simulink model "l512_devel_pps_2016f"  (R2012b)
settings: Solver=ode45  StartTime=0.0  StopTime=15000  RelTol=1e-3
undefined symbols (not defined in the file): sfp
libraries: xbsIndex_r4 x7383, casper_library_misc x259, casper_library_delays x118, xps_library x12, simulink x1
(part 3 of 82)

== system l512_devel_pps_2016f/fft ==
  In1 : Inport
  f1 : Subsystem
  f2 : Subsystem
  f3 : Subsystem
  f4 : Subsystem
  Out2 : Outport
  tag scope: eq_out1=global, eq_out2=global, eq_out3=global, eq_out=global, sync_rnd1=global, sync_rnd2=global, sync_rnd3=global, sync_rnd=global
  wires:
  In1/1 -> Out2/1
  [adc0] -> f1/1(adc1)
  [adc1] -> f1/2(adc2)
  f1/2(eq_out) -> [eq_out]
  [adc2] -> f1/3(adc3)
  [adc3] -> f1/4(adc4)
  [adc4] -> f1/5(adc5)
  [adc5] -> f1/6(adc6)
  [adc6] -> f1/7(adc7)
  [adc7] -> f1/8(adc8)
  f3/2(eq_out) -> [eq_out2]
  f3/1(sync_rnd1) -> [sync_rnd2]
  f2/2(eq_out) -> [eq_out1]
  f2/1(sync_rnd1) -> [sync_rnd1]
  f1/1(sync_rnd1) -> [sync_rnd]
  [adc10] -> f2/3(adc3)
  [adc14] -> f2/7(adc7)
  [adc11] -> f2/4(adc4)
  [adc12] -> f2/5(adc5)
  [adc13] -> f2/6(adc6)
  [adc8] -> f2/1(adc1)
  [adc15] -> f2/8(adc8)
  [adc9] -> f2/2(adc2)
  [adc21] -> f3/6(adc6)
  [adc22] -> f3/7(adc7)
  [adc23] -> f3/8(adc8)
  [adc18] -> f3/3(adc3)
  [adc19] -> f3/4(adc4)
  [adc20] -> f3/5(adc5)
  [adc17] -> f3/2(adc2)
  [adc16] -> f3/1(adc1)
  [adc25] -> f4/2(adc2)
  [adc24] -> f4/1(adc1)
  [adc29] -> f4/6(adc6)
  [adc26] -> f4/3(adc3)
  [adc27] -> f4/4(adc4)
  [adc28] -> f4/5(adc5)
  [adc30] -> f4/7(adc7)
  [adc31] -> f4/8(adc8)
  f4/1(sync_rnd1) -> [sync_rnd3]
  f4/2(eq_out) -> [eq_out3]
